simulink model "ServoControl"  (R2014a)
settings: Solver=ode45  StartTime=0.0  StopTime=2000000  RelTol=1e-3
libraries: hdlsllib x2, simulink x1
settings Model: Creator=amir  LastModifiedBy=Shiyu
settings OptimizationCC: BlockReduction=off  ConditionallyExecuteInputs=off  InlineParams=on
settings DebuggingCC: AlgebraicLoopMsg=error  MergeDetectMultiDrivingBlocksExec=error  IntegerOverflowMsg=none  ParameterOverflowMsg=none
settings HardwareCC: ProdHWDeviceType=ASIC/FPGA->ASIC/FPGA  ProdEqTarget=off

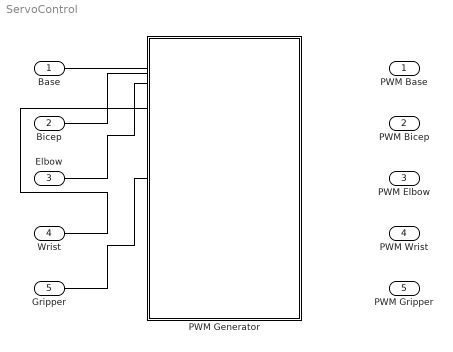
== system ServoControl ==
  Base : Inport  OutDataTypeStr=uint8  SampleTime=1
  Bicep : Inport  Port=2  OutDataTypeStr=uint8  SampleTime=1
  Elbow : Inport  Port=3  OutDataTypeStr=uint8  SampleTime=1
  Wrist : Inport  Port=4  OutDataTypeStr=uint8  SampleTime=1
  Gripper : Inport  Port=5  OutDataTypeStr=uint8  SampleTime=1
  PWM Generator : Subsystem  TreatAsAtomicUnit=on
  PWM Base : Outport
  PWM Bicep : Outport  Port=2
  PWM Elbow : Outport  Port=3
  PWM Wrist : Outport  Port=4
  PWM Gripper : Outport  Port=5
  wires:
  Base/1 -> ?
  Bicep/1 -> ?
  Elbow/1 -> ?
  Wrist/1 -> ?
  Gripper/1 -> ?
  ? -> PWM Base/1
  ? -> PWM Bicep/1
  ? -> PWM Elbow/1
  ? -> PWM Wrist/1
  ? -> PWM Gripper/1

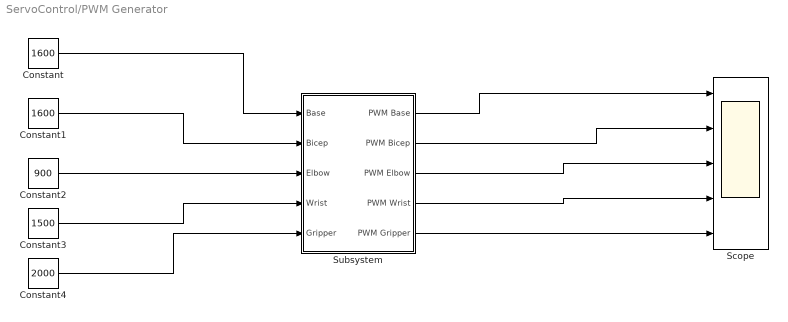
== system ServoControl/PWM Generator ==
  Constant : Constant  Value=1600  OutDataTypeStr=uint8
  Constant1 : Constant  Value=1600  OutDataTypeStr=uint8
  Constant2 : Constant  Value=900  OutDataTypeStr=uint8
  Constant3 : Constant  Value=1500  OutDataTypeStr=uint8
  Constant4 : Constant  Value=2000  OutDataTypeStr=uint8
  Scope : Scope  NumInputPorts=5
      settings: TimeRange=200000  YMin=0~0~0~0~0  YMax=1~1~1~1~1
  Subsystem : Subsystem
  wires:
  Constant/1 -> Subsystem/1(Base)
  Constant1/1 -> Subsystem/2(Bicep)
  Constant2/1 -> Subsystem/3(Elbow)
  Constant3/1 -> Subsystem/4(Wrist)
  Constant4/1 -> Subsystem/5(Gripper)
  Subsystem/1(PWM Base) -> Scope/1
  Subsystem/2(PWM Bicep) -> Scope/2
  Subsystem/3(PWM Elbow) -> Scope/3
  Subsystem/4(PWM Wrist) -> Scope/4
  Subsystem/5(PWM Gripper) -> Scope/5

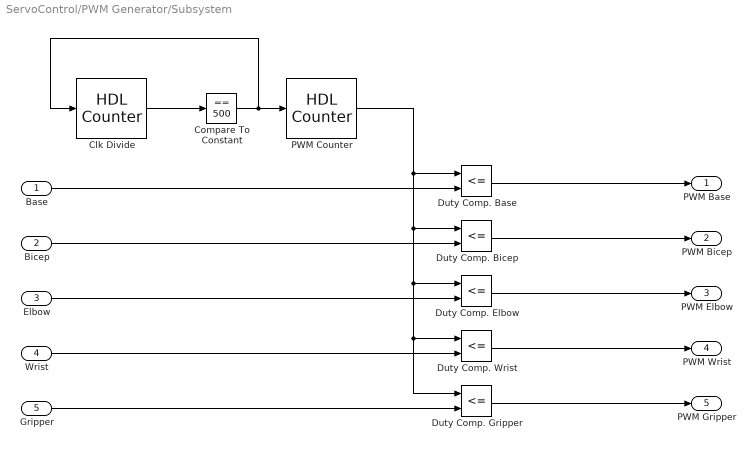
== system ServoControl/PWM Generator/Subsystem ==
  Base : Inport  OutDataTypeStr=uint8  SampleTime=1
  Bicep : Inport  Port=2  OutDataTypeStr=uint8  SampleTime=1
  Elbow : Inport  Port=3  OutDataTypeStr=uint8  SampleTime=1
  Wrist : Inport  Port=4  OutDataTypeStr=uint8  SampleTime=1
  Gripper : Inport  Port=5  OutDataTypeStr=uint8  SampleTime=1
  Clk Divide : hdlsllib/HDL Operations/HDL Counter  CountType=Free running  CountInit=1  CountStep=1  CountMax=500  CountFromType=Initial value  CountFrom=1  CountResetPort=on  CountLoadPort=off  CountEnbPort=off  CountDirPort=off  CountDataType=Unsigned  CountWordLen=16  CountFracLen=0  CountSampTime=1
  Compare To Constant : simulink/Logic and Bit Operations/Compare To Constant  relop===  const=500  OutDataTypeStr=boolean
  Duty Comp. Base : RelationalOperator  Operator=<=  OutDataTypeStr=boolean
  Duty Comp. Bicep : RelationalOperator  Operator=<=  OutDataTypeStr=boolean
  Duty Comp. Elbow : RelationalOperator  Operator=<=  OutDataTypeStr=boolean
  Duty Comp. Gripper : RelationalOperator  Operator=<=  OutDataTypeStr=boolean
  Duty Comp. Wrist : RelationalOperator  Operator=<=  OutDataTypeStr=boolean
  PWM Counter : hdlsllib/HDL Operations/HDL Counter  CountType=Count limited  CountInit=1  CountStep=1  CountMax=2000  CountFromType=Initial value  CountFrom=1  CountResetPort=off  CountLoadPort=off  CountEnbPort=on  CountDirPort=off  CountDataType=Unsigned  CountWordLen=16  CountFracLen=0  CountSampTime=1
  PWM Base : Outport
  PWM Bicep : Outport  Port=2
  PWM Elbow : Outport  Port=3
  PWM Wrist : Outport  Port=4
  PWM Gripper : Outport  Port=5
  wires:
  Elbow/1 -> Duty Comp. Elbow/2
  Clk Divide/1 -> Compare To Constant/1
  Compare To Constant/1 -> Clk Divide/1, PWM Counter/1
  Gripper/1 -> Duty Comp. Gripper/2
  Duty Comp. Gripper/1 -> PWM Gripper/1
  Wrist/1 -> Duty Comp. Wrist/2
  Base/1 -> Duty Comp. Base/2
  Duty Comp. Bicep/1 -> PWM Bicep/1
  Duty Comp. Elbow/1 -> PWM Elbow/1
  Duty Comp. Wrist/1 -> PWM Wrist/1
  Duty Comp. Base/1 -> PWM Base/1
  PWM Counter/1 -> Duty Comp. Base/1, Duty Comp. Bicep/1, Duty Comp. Elbow/1, Duty Comp. Wrist/1, Duty Comp. Gripper/1
  Bicep/1 -> Duty Comp. Bicep/2
